simulink model "building_EXAMPLE_v1"  (R2016b)
settings: Solver=ode23tb  StartTime=-building.preruntime+8760*3600  StopTime=building.runtime+8760*3600  MaxStep=600  EnableMultiTasking=on
StartFcn:
  | tic
StopFcn:
  | toc
values from neighbouring files (symbols this model uses):
  building = create_building_automatic(building, modify, import_mode, name_XML, name_EXCEL, name_PHPP, NUMBEROFZONES)    [work_EXAMPLE_v1.m]
undefined symbols (not defined in the file or in its folder): A, B, C, cp, Dd, Dreifach, FluidMix, get_building, ID, MassFlow, p, Pressure, Qdot_C, Qdot_C_energy, Qdot_H, Qdot_H_energy, Qdot_I_electricity, Qdot_I_electricity_energy, Qdot_I_light, Qdot_I_light_energy, Qdot_I_person, Qdot_I_person_energy, Qdot_S, Qdot_S_energy, Qdot_T_ground, Qdot_T_ground_energy, Qdot_T_neighbour, Qdot_T_neighbour_energy, Qdot_T_opaque, Qdot_T_opaque_energy, Qdot_T_window, Qdot_T_window_energy, Qdot_V_infiltration, Qdot_V_infiltration_energy, Qdot_V_mech, Qdot_V_mech_energy, Qdot_V_window, Qdot_V_window_energy, rho, Tc, Temperature, Tr, Ts, Wärmeschutzglas, x_CO2, x_H2O, x_VOC
libraries: carnotUIBK x1931, carnot x83, simulink_extras x22, simulink x12
(part 12 of 35)

== system building_EXAMPLE_v1/HVAC pipes/ventilation_outlet1_z10 ==
  note: see energy balance
  note: no energy flux
  "[AIB]" : Inport
  Vdot : Inport  Port=2
  (kg/m³).(m³/h) : Product
  Bus Selector1 : BusSelector  OutputSignals=rho,Tc,p
  Bus Selector2 : BusSelector  OutputSignals=x_H2O
  Bus Selector3 : BusSelector  OutputSignals=x_CO2
  Fcn1 : Fcn  Expr=u / (1+u)
  Fcn2 : Fcn  Expr=u / (1+u)
  Gain : Gain  Gain=perc_Vdot_tot
  Gain1 : Gain  Gain=-1
  Gain3 : Gain  Gain=-1
  Gain4 : Gain  Gain=-1
  Ground{1..5} (5 alike) : Ground
  Mux1 : Mux  Inputs=[1 2 1 1 1 5 1 7]
  create_THB : Subsystem  mask(create THV){fluid=2, dia=0.125, hgt=0, mID=1}
      mask prompts: dia "diameter [m]"; hgt "Geodetic height in m"; mID "Calculation mode"
      mask help:
      | Create a THB with the variable input T and mdot. The other value can be set as constants in the mask.
      | Calculation mode:
      |     1 ..  9999 no pressure drop (dp)
      | 10001 .. 19999 dp caused by flowrate
      | 20001 .. inf   dp by flowrate and static height
      mask init:
      | dia = max(dia, 0.001);
      mask Help: web(fullfile(path_carnot('help'),'basic_create_THB.html'),'-helpbrowser')
  h/s : Gain  Gain=1/3600
  kg/s : Product
  kg/s1 : Product
  "[S]" : Outport
  THBout : Outport  Port=2  InitialOutput=0
  wires:
  create_THB/1(THB) -> THBout/1
  Bus Selector1/3 -> create_THB/3(p)  "<p>"
  Bus Selector1/2 -> create_THB/2(T)  "<Tc>"
  Vdot/1 -> Gain/1
  Ground3/1 -> Mux1/2
  Ground2/1 -> Mux1/8
  Ground1/1 -> Mux1/7
  Bus Selector3/1 -> Fcn1/1  "<x_CO2>"
  Bus Selector1/1 -> (kg/m³).(m³/h)/1  "<rho>"
  "[AIB]"/1 -> Bus Selector2/1, Bus Selector3/1, Bus Selector1/1
  Gain1/1 -> Mux1/5
  kg/s1/1 -> Gain1/1
  Fcn1/1 -> kg/s1/2
  Fcn2/1 -> kg/s/2
  Gain4/1 -> Mux1/3
  Ground5/1 -> Mux1/6
  Ground4/1 -> Mux1/1
  Gain3/1 -> Mux1/4
  kg/s/1 -> Gain3/1
  Bus Selector2/1 -> create_THB/4(mix), Fcn2/1  "<x_H2O>"
  h/s/1 -> Gain4/1, kg/s/1, create_THB/1(mdot), kg/s1/1
  (kg/m³).(m³/h)/1 -> h/s/1
  Gain/1 -> (kg/m³).(m³/h)/2
  Mux1/1 -> "[S]"/1

== system building_EXAMPLE_v1/HVAC pipes/ventilation_outlet1_z2 ==
  note: see energy balance
  note: no energy flux
  "[AIB]" : Inport
  Vdot : Inport  Port=2
  (kg/m³).(m³/h) : Product
  Bus Selector1 : BusSelector  OutputSignals=rho,Tc,p
  Bus Selector2 : BusSelector  OutputSignals=x_H2O
  Bus Selector3 : BusSelector  OutputSignals=x_CO2
  Fcn1 : Fcn  Expr=u / (1+u)
  Fcn2 : Fcn  Expr=u / (1+u)
  Gain : Gain  Gain=perc_Vdot_tot
  Gain1 : Gain  Gain=-1
  Gain3 : Gain  Gain=-1
  Gain4 : Gain  Gain=-1
  Ground{1..5} (5 alike) : Ground
  Mux1 : Mux  Inputs=[1 2 1 1 1 5 1 7]
  create_THB : Subsystem  mask(create THV){fluid=2, dia=0.125, hgt=0, mID=1}
      mask prompts: dia "diameter [m]"; hgt "Geodetic height in m"; mID "Calculation mode"
      mask help:
      | Create a THB with the variable input T and mdot. The other value can be set as constants in the mask.
      | Calculation mode:
      |     1 ..  9999 no pressure drop (dp)
      | 10001 .. 19999 dp caused by flowrate
      | 20001 .. inf   dp by flowrate and static height
      mask init:
      | dia = max(dia, 0.001);
      mask Help: web(fullfile(path_carnot('help'),'basic_create_THB.html'),'-helpbrowser')
  h/s : Gain  Gain=1/3600
  kg/s : Product
  kg/s1 : Product
  "[S]" : Outport
  THBout : Outport  Port=2  InitialOutput=0
  wires:
  create_THB/1(THB) -> THBout/1
  Bus Selector1/3 -> create_THB/3(p)  "<p>"
  Bus Selector1/2 -> create_THB/2(T)  "<Tc>"
  Vdot/1 -> Gain/1
  Ground3/1 -> Mux1/2
  Ground2/1 -> Mux1/8
  Ground1/1 -> Mux1/7
  Bus Selector3/1 -> Fcn1/1  "<x_CO2>"
  Bus Selector1/1 -> (kg/m³).(m³/h)/1  "<rho>"
  "[AIB]"/1 -> Bus Selector2/1, Bus Selector3/1, Bus Selector1/1
  Gain1/1 -> Mux1/5
  kg/s1/1 -> Gain1/1
  Fcn1/1 -> kg/s1/2
  Fcn2/1 -> kg/s/2
  Gain4/1 -> Mux1/3
  Ground5/1 -> Mux1/6
  Ground4/1 -> Mux1/1
  Gain3/1 -> Mux1/4
  kg/s/1 -> Gain3/1
  Bus Selector2/1 -> create_THB/4(mix), Fcn2/1  "<x_H2O>"
  h/s/1 -> Gain4/1, kg/s/1, create_THB/1(mdot), kg/s1/1
  (kg/m³).(m³/h)/1 -> h/s/1
  Gain/1 -> (kg/m³).(m³/h)/2
  Mux1/1 -> "[S]"/1

== system building_EXAMPLE_v1/HVAC pipes/ventilation_outlet1_z3 ==
  note: no energy flux
  note: see energy balance
  "[AIB]" : Inport
  Vdot : Inport  Port=2
  (kg/m³).(m³/h) : Product
  Bus Selector1 : BusSelector  OutputSignals=rho,Tc,p
  Bus Selector2 : BusSelector  OutputSignals=x_H2O
  Bus Selector3 : BusSelector  OutputSignals=x_CO2
  Fcn1 : Fcn  Expr=u / (1+u)
  Fcn2 : Fcn  Expr=u / (1+u)
  Gain : Gain  Gain=perc_Vdot_tot
  Gain1 : Gain  Gain=-1
  Gain3 : Gain  Gain=-1
  Gain4 : Gain  Gain=-1
  Ground{1..5} (5 alike) : Ground
  Mux1 : Mux  Inputs=[1 2 1 1 1 5 1 7]
  create_THB : Subsystem  mask(create THV){fluid=2, dia=0.125, hgt=0, mID=1}
      mask prompts: dia "diameter [m]"; hgt "Geodetic height in m"; mID "Calculation mode"
      mask help:
      | Create a THB with the variable input T and mdot. The other value can be set as constants in the mask.
      | Calculation mode:
      |     1 ..  9999 no pressure drop (dp)
      | 10001 .. 19999 dp caused by flowrate
      | 20001 .. inf   dp by flowrate and static height
      mask init:
      | dia = max(dia, 0.001);
      mask Help: web(fullfile(path_carnot('help'),'basic_create_THB.html'),'-helpbrowser')
  h/s : Gain  Gain=1/3600
  kg/s : Product
  kg/s1 : Product
  "[S]" : Outport
  THBout : Outport  Port=2  InitialOutput=0
  wires:
  Mux1/1 -> "[S]"/1
  Gain/1 -> (kg/m³).(m³/h)/2
  (kg/m³).(m³/h)/1 -> h/s/1
  h/s/1 -> create_THB/1(mdot), kg/s1/1, kg/s/1, Gain4/1
  Bus Selector2/1 -> create_THB/4(mix), Fcn2/1  "<x_H2O>"
  kg/s/1 -> Gain3/1
  Gain3/1 -> Mux1/4
  Ground4/1 -> Mux1/1
  Ground5/1 -> Mux1/6
  Gain4/1 -> Mux1/3
  Fcn2/1 -> kg/s/2
  Fcn1/1 -> kg/s1/2
  kg/s1/1 -> Gain1/1
  Gain1/1 -> Mux1/5
  "[AIB]"/1 -> Bus Selector1/1, Bus Selector3/1, Bus Selector2/1
  Bus Selector1/1 -> (kg/m³).(m³/h)/1  "<rho>"
  Bus Selector3/1 -> Fcn1/1  "<x_CO2>"
  Ground1/1 -> Mux1/7
  Ground2/1 -> Mux1/8
  Ground3/1 -> Mux1/2
  Vdot/1 -> Gain/1
  Bus Selector1/2 -> create_THB/2(T)  "<Tc>"
  Bus Selector1/3 -> create_THB/3(p)  "<p>"
  create_THB/1(THB) -> THBout/1

== system building_EXAMPLE_v1/HVAC pipes/ventilation_outlet1_z4 ==
  note: see energy balance
  note: no energy flux
  "[AIB]" : Inport
  Vdot : Inport  Port=2
  (kg/m³).(m³/h) : Product
  Bus Selector1 : BusSelector  OutputSignals=rho,Tc,p
  Bus Selector2 : BusSelector  OutputSignals=x_H2O
  Bus Selector3 : BusSelector  OutputSignals=x_CO2
  Fcn1 : Fcn  Expr=u / (1+u)
  Fcn2 : Fcn  Expr=u / (1+u)
  Gain : Gain  Gain=perc_Vdot_tot
  Gain1 : Gain  Gain=-1
  Gain3 : Gain  Gain=-1
  Gain4 : Gain  Gain=-1
  Ground{1..5} (5 alike) : Ground
  Mux1 : Mux  Inputs=[1 2 1 1 1 5 1 7]
  create_THB : Subsystem  mask(create THV){fluid=2, dia=0.125, hgt=0, mID=1}
      mask prompts: dia "diameter [m]"; hgt "Geodetic height in m"; mID "Calculation mode"
      mask help:
      | Create a THB with the variable input T and mdot. The other value can be set as constants in the mask.
      | Calculation mode:
      |     1 ..  9999 no pressure drop (dp)
      | 10001 .. 19999 dp caused by flowrate
      | 20001 .. inf   dp by flowrate and static height
      mask init:
      | dia = max(dia, 0.001);
      mask Help: web(fullfile(path_carnot('help'),'basic_create_THB.html'),'-helpbrowser')
  h/s : Gain  Gain=1/3600
  kg/s : Product
  kg/s1 : Product
  "[S]" : Outport
  THBout : Outport  Port=2  InitialOutput=0
  wires:
  create_THB/1(THB) -> THBout/1
  Bus Selector1/3 -> create_THB/3(p)  "<p>"
  Bus Selector1/2 -> create_THB/2(T)  "<Tc>"
  Vdot/1 -> Gain/1
  Ground3/1 -> Mux1/2
  Ground2/1 -> Mux1/8
  Ground1/1 -> Mux1/7
  Bus Selector3/1 -> Fcn1/1  "<x_CO2>"
  Bus Selector1/1 -> (kg/m³).(m³/h)/1  "<rho>"
  "[AIB]"/1 -> Bus Selector2/1, Bus Selector3/1, Bus Selector1/1
  Gain1/1 -> Mux1/5
  kg/s1/1 -> Gain1/1
  Fcn1/1 -> kg/s1/2
  Fcn2/1 -> kg/s/2
  Gain4/1 -> Mux1/3
  Ground5/1 -> Mux1/6
  Ground4/1 -> Mux1/1
  Gain3/1 -> Mux1/4
  kg/s/1 -> Gain3/1
  Bus Selector2/1 -> create_THB/4(mix), Fcn2/1  "<x_H2O>"
  h/s/1 -> Gain4/1, kg/s/1, create_THB/1(mdot), kg/s1/1
  (kg/m³).(m³/h)/1 -> h/s/1
  Gain/1 -> (kg/m³).(m³/h)/2
  Mux1/1 -> "[S]"/1

== system building_EXAMPLE_v1/HVAC pipes/ventilation_outlet1_z5 ==
  note: no energy flux
  note: see energy balance
  "[AIB]" : Inport
  Vdot : Inport  Port=2
  (kg/m³).(m³/h) : Product
  Bus Selector1 : BusSelector  OutputSignals=rho,Tc,p
  Bus Selector2 : BusSelector  OutputSignals=x_H2O
  Bus Selector3 : BusSelector  OutputSignals=x_CO2
  Fcn1 : Fcn  Expr=u / (1+u)
  Fcn2 : Fcn  Expr=u / (1+u)
  Gain : Gain  Gain=perc_Vdot_tot
  Gain1 : Gain  Gain=-1
  Gain3 : Gain  Gain=-1
  Gain4 : Gain  Gain=-1
  Ground{1..5} (5 alike) : Ground
  Mux1 : Mux  Inputs=[1 2 1 1 1 5 1 7]
  create_THB : Subsystem  mask(create THV){fluid=2, dia=0.125, hgt=0, mID=1}
      mask prompts: dia "diameter [m]"; hgt "Geodetic height in m"; mID "Calculation mode"
      mask help:
      | Create a THB with the variable input T and mdot. The other value can be set as constants in the mask.
      | Calculation mode:
      |     1 ..  9999 no pressure drop (dp)
      | 10001 .. 19999 dp caused by flowrate
      | 20001 .. inf   dp by flowrate and static height
      mask init:
      | dia = max(dia, 0.001);
      mask Help: web(fullfile(path_carnot('help'),'basic_create_THB.html'),'-helpbrowser')
  h/s : Gain  Gain=1/3600
  kg/s : Product
  kg/s1 : Product
  "[S]" : Outport
  THBout : Outport  Port=2  InitialOutput=0
  wires:
  Mux1/1 -> "[S]"/1
  Gain/1 -> (kg/m³).(m³/h)/2
  (kg/m³).(m³/h)/1 -> h/s/1
  h/s/1 -> create_THB/1(mdot), kg/s1/1, kg/s/1, Gain4/1
  Bus Selector2/1 -> create_THB/4(mix), Fcn2/1  "<x_H2O>"
  kg/s/1 -> Gain3/1
  Gain3/1 -> Mux1/4
  Ground4/1 -> Mux1/1
  Ground5/1 -> Mux1/6
  Gain4/1 -> Mux1/3
  Fcn2/1 -> kg/s/2
  Fcn1/1 -> kg/s1/2
  kg/s1/1 -> Gain1/1
  Gain1/1 -> Mux1/5
  "[AIB]"/1 -> Bus Selector1/1, Bus Selector3/1, Bus Selector2/1
  Bus Selector1/1 -> (kg/m³).(m³/h)/1  "<rho>"
  Bus Selector3/1 -> Fcn1/1  "<x_CO2>"
  Ground1/1 -> Mux1/7
  Ground2/1 -> Mux1/8
  Ground3/1 -> Mux1/2
  Vdot/1 -> Gain/1
  Bus Selector1/2 -> create_THB/2(T)  "<Tc>"
  Bus Selector1/3 -> create_THB/3(p)  "<p>"
  create_THB/1(THB) -> THBout/1

== system building_EXAMPLE_v1/HVAC pipes/ventilation_outlet1_z6 ==
  note: see energy balance
  note: no energy flux
  "[AIB]" : Inport
  Vdot : Inport  Port=2
  (kg/m³).(m³/h) : Product
  Bus Selector1 : BusSelector  OutputSignals=rho,Tc,p
  Bus Selector2 : BusSelector  OutputSignals=x_H2O
  Bus Selector3 : BusSelector  OutputSignals=x_CO2
  Fcn1 : Fcn  Expr=u / (1+u)
  Fcn2 : Fcn  Expr=u / (1+u)
  Gain : Gain  Gain=perc_Vdot_tot
  Gain1 : Gain  Gain=-1
  Gain3 : Gain  Gain=-1
  Gain4 : Gain  Gain=-1
  Ground{1..5} (5 alike) : Ground
  Mux1 : Mux  Inputs=[1 2 1 1 1 5 1 7]
  create_THB : Subsystem  mask(create THV){fluid=2, dia=0.125, hgt=0, mID=1}
      mask prompts: dia "diameter [m]"; hgt "Geodetic height in m"; mID "Calculation mode"
      mask help:
      | Create a THB with the variable input T and mdot. The other value can be set as constants in the mask.
      | Calculation mode:
      |     1 ..  9999 no pressure drop (dp)
      | 10001 .. 19999 dp caused by flowrate
      | 20001 .. inf   dp by flowrate and static height
      mask init:
      | dia = max(dia, 0.001);
      mask Help: web(fullfile(path_carnot('help'),'basic_create_THB.html'),'-helpbrowser')
  h/s : Gain  Gain=1/3600
  kg/s : Product
  kg/s1 : Product
  "[S]" : Outport
  THBout : Outport  Port=2  InitialOutput=0
  wires:
  create_THB/1(THB) -> THBout/1
  Bus Selector1/3 -> create_THB/3(p)  "<p>"
  Bus Selector1/2 -> create_THB/2(T)  "<Tc>"
  Vdot/1 -> Gain/1
  Ground3/1 -> Mux1/2
  Ground2/1 -> Mux1/8
  Ground1/1 -> Mux1/7
  Bus Selector3/1 -> Fcn1/1  "<x_CO2>"
  Bus Selector1/1 -> (kg/m³).(m³/h)/1  "<rho>"
  "[AIB]"/1 -> Bus Selector2/1, Bus Selector3/1, Bus Selector1/1
  Gain1/1 -> Mux1/5
  kg/s1/1 -> Gain1/1
  Fcn1/1 -> kg/s1/2
  Fcn2/1 -> kg/s/2
  Gain4/1 -> Mux1/3
  Ground5/1 -> Mux1/6
  Ground4/1 -> Mux1/1
  Gain3/1 -> Mux1/4
  kg/s/1 -> Gain3/1
  Bus Selector2/1 -> create_THB/4(mix), Fcn2/1  "<x_H2O>"
  h/s/1 -> Gain4/1, kg/s/1, create_THB/1(mdot), kg/s1/1
  (kg/m³).(m³/h)/1 -> h/s/1
  Gain/1 -> (kg/m³).(m³/h)/2
  Mux1/1 -> "[S]"/1

== system building_EXAMPLE_v1/HVAC pipes/ventilation_outlet1_z7 ==
  note: no energy flux
  note: see energy balance
  "[AIB]" : Inport
  Vdot : Inport  Port=2
  (kg/m³).(m³/h) : Product
  Bus Selector1 : BusSelector  OutputSignals=rho,Tc,p
  Bus Selector2 : BusSelector  OutputSignals=x_H2O
  Bus Selector3 : BusSelector  OutputSignals=x_CO2
  Fcn1 : Fcn  Expr=u / (1+u)
  Fcn2 : Fcn  Expr=u / (1+u)
  Gain : Gain  Gain=perc_Vdot_tot
  Gain1 : Gain  Gain=-1
  Gain3 : Gain  Gain=-1
  Gain4 : Gain  Gain=-1
  Ground{1..5} (5 alike) : Ground
  Mux1 : Mux  Inputs=[1 2 1 1 1 5 1 7]
  create_THB : Subsystem  mask(create THV){fluid=2, dia=0.125, hgt=0, mID=1}
      mask prompts: dia "diameter [m]"; hgt "Geodetic height in m"; mID "Calculation mode"
      mask help:
      | Create a THB with the variable input T and mdot. The other value can be set as constants in the mask.
      | Calculation mode:
      |     1 ..  9999 no pressure drop (dp)
      | 10001 .. 19999 dp caused by flowrate
      | 20001 .. inf   dp by flowrate and static height
      mask init:
      | dia = max(dia, 0.001);
      mask Help: web(fullfile(path_carnot('help'),'basic_create_THB.html'),'-helpbrowser')
  h/s : Gain  Gain=1/3600
  kg/s : Product
  kg/s1 : Product
  "[S]" : Outport
  THBout : Outport  Port=2  InitialOutput=0
  wires:
  Mux1/1 -> "[S]"/1
  Gain/1 -> (kg/m³).(m³/h)/2
  (kg/m³).(m³/h)/1 -> h/s/1
  h/s/1 -> create_THB/1(mdot), kg/s1/1, kg/s/1, Gain4/1
  Bus Selector2/1 -> create_THB/4(mix), Fcn2/1  "<x_H2O>"
  kg/s/1 -> Gain3/1
  Gain3/1 -> Mux1/4
  Ground4/1 -> Mux1/1
  Ground5/1 -> Mux1/6
  Gain4/1 -> Mux1/3
  Fcn2/1 -> kg/s/2
  Fcn1/1 -> kg/s1/2
  kg/s1/1 -> Gain1/1
  Gain1/1 -> Mux1/5
  "[AIB]"/1 -> Bus Selector1/1, Bus Selector3/1, Bus Selector2/1
  Bus Selector1/1 -> (kg/m³).(m³/h)/1  "<rho>"
  Bus Selector3/1 -> Fcn1/1  "<x_CO2>"
  Ground1/1 -> Mux1/7
  Ground2/1 -> Mux1/8
  Ground3/1 -> Mux1/2
  Vdot/1 -> Gain/1
  Bus Selector1/2 -> create_THB/2(T)  "<Tc>"
  Bus Selector1/3 -> create_THB/3(p)  "<p>"
  create_THB/1(THB) -> THBout/1

== system building_EXAMPLE_v1/HVAC pipes/ventilation_outlet1_z8 ==
  note: see energy balance
  note: no energy flux
  "[AIB]" : Inport
  Vdot : Inport  Port=2
  (kg/m³).(m³/h) : Product
  Bus Selector1 : BusSelector  OutputSignals=rho,Tc,p
  Bus Selector2 : BusSelector  OutputSignals=x_H2O
  Bus Selector3 : BusSelector  OutputSignals=x_CO2
  Fcn1 : Fcn  Expr=u / (1+u)
  Fcn2 : Fcn  Expr=u / (1+u)
  Gain : Gain  Gain=perc_Vdot_tot
  Gain1 : Gain  Gain=-1
  Gain3 : Gain  Gain=-1
  Gain4 : Gain  Gain=-1
  Ground{1..5} (5 alike) : Ground
  Mux1 : Mux  Inputs=[1 2 1 1 1 5 1 7]
  create_THB : Subsystem  mask(create THV){fluid=2, dia=0.125, hgt=0, mID=1}
      mask prompts: dia "diameter [m]"; hgt "Geodetic height in m"; mID "Calculation mode"
      mask help:
      | Create a THB with the variable input T and mdot. The other value can be set as constants in the mask.
      | Calculation mode:
      |     1 ..  9999 no pressure drop (dp)
      | 10001 .. 19999 dp caused by flowrate
      | 20001 .. inf   dp by flowrate and static height
      mask init:
      | dia = max(dia, 0.001);
      mask Help: web(fullfile(path_carnot('help'),'basic_create_THB.html'),'-helpbrowser')
  h/s : Gain  Gain=1/3600
  kg/s : Product
  kg/s1 : Product
  "[S]" : Outport
  THBout : Outport  Port=2  InitialOutput=0
  wires:
  create_THB/1(THB) -> THBout/1
  Bus Selector1/3 -> create_THB/3(p)  "<p>"
  Bus Selector1/2 -> create_THB/2(T)  "<Tc>"
  Vdot/1 -> Gain/1
  Ground3/1 -> Mux1/2
  Ground2/1 -> Mux1/8
  Ground1/1 -> Mux1/7
  Bus Selector3/1 -> Fcn1/1  "<x_CO2>"
  Bus Selector1/1 -> (kg/m³).(m³/h)/1  "<rho>"
  "[AIB]"/1 -> Bus Selector2/1, Bus Selector3/1, Bus Selector1/1
  Gain1/1 -> Mux1/5
  kg/s1/1 -> Gain1/1
  Fcn1/1 -> kg/s1/2
  Fcn2/1 -> kg/s/2
  Gain4/1 -> Mux1/3
  Ground5/1 -> Mux1/6
  Ground4/1 -> Mux1/1
  Gain3/1 -> Mux1/4
  kg/s/1 -> Gain3/1
  Bus Selector2/1 -> create_THB/4(mix), Fcn2/1  "<x_H2O>"
  h/s/1 -> Gain4/1, kg/s/1, create_THB/1(mdot), kg/s1/1
  (kg/m³).(m³/h)/1 -> h/s/1
  Gain/1 -> (kg/m³).(m³/h)/2
  Mux1/1 -> "[S]"/1

== system building_EXAMPLE_v1/HVAC pipes/ventilation_outlet1_z9 ==
  note: no energy flux
  note: see energy balance
  "[AIB]" : Inport
  Vdot : Inport  Port=2
  (kg/m³).(m³/h) : Product
  Bus Selector1 : BusSelector  OutputSignals=rho,Tc,p
  Bus Selector2 : BusSelector  OutputSignals=x_H2O
  Bus Selector3 : BusSelector  OutputSignals=x_CO2
  Fcn1 : Fcn  Expr=u / (1+u)
  Fcn2 : Fcn  Expr=u / (1+u)
  Gain : Gain  Gain=perc_Vdot_tot
  Gain1 : Gain  Gain=-1
  Gain3 : Gain  Gain=-1
  Gain4 : Gain  Gain=-1
  Ground{1..5} (5 alike) : Ground
  Mux1 : Mux  Inputs=[1 2 1 1 1 5 1 7]
  create_THB : Subsystem  mask(create THV){fluid=2, dia=0.125, hgt=0, mID=1}
      mask prompts: dia "diameter [m]"; hgt "Geodetic height in m"; mID "Calculation mode"
      mask help:
      | Create a THB with the variable input T and mdot. The other value can be set as constants in the mask.
      | Calculation mode:
      |     1 ..  9999 no pressure drop (dp)
      | 10001 .. 19999 dp caused by flowrate
      | 20001 .. inf   dp by flowrate and static height
      mask init:
      | dia = max(dia, 0.001);
      mask Help: web(fullfile(path_carnot('help'),'basic_create_THB.html'),'-helpbrowser')
  h/s : Gain  Gain=1/3600
  kg/s : Product
  kg/s1 : Product
  "[S]" : Outport
  THBout : Outport  Port=2  InitialOutput=0
  wires:
  Mux1/1 -> "[S]"/1
  Gain/1 -> (kg/m³).(m³/h)/2
  (kg/m³).(m³/h)/1 -> h/s/1
  h/s/1 -> create_THB/1(mdot), kg/s1/1, kg/s/1, Gain4/1
  Bus Selector2/1 -> create_THB/4(mix), Fcn2/1  "<x_H2O>"
  kg/s/1 -> Gain3/1
  Gain3/1 -> Mux1/4
  Ground4/1 -> Mux1/1
  Ground5/1 -> Mux1/6
  Gain4/1 -> Mux1/3
  Fcn2/1 -> kg/s/2
  Fcn1/1 -> kg/s1/2
  kg/s1/1 -> Gain1/1
  Gain1/1 -> Mux1/5
  "[AIB]"/1 -> Bus Selector1/1, Bus Selector3/1, Bus Selector2/1
  Bus Selector1/1 -> (kg/m³).(m³/h)/1  "<rho>"
  Bus Selector3/1 -> Fcn1/1  "<x_CO2>"
  Ground1/1 -> Mux1/7
  Ground2/1 -> Mux1/8
  Ground3/1 -> Mux1/2
  Vdot/1 -> Gain/1
  Bus Selector1/2 -> create_THB/2(T)  "<Tc>"
  Bus Selector1/3 -> create_THB/3(p)  "<p>"
  create_THB/1(THB) -> THBout/1

== system building_EXAMPLE_v1/HVAC pipes/ventilation_pipe_in_1 ==
  THBsupply : Inport
  Bus Selector : BusSelector  OutputSignals=MassFlow
  THB_set_mdot{1..10} (10 alike) : carnot/Source/Simple/THB_set_mdot
  zone_1 : Gain  Gain=hvac.zone(1).inlet(1)
  zone_10 : Gain  Gain=hvac.zone(10).inlet(1)
  zone_2 : Gain  Gain=hvac.zone(2).inlet(1)
  zone_3 : Gain  Gain=hvac.zone(3).inlet(1)
  zone_4 : Gain  Gain=hvac.zone(4).inlet(1)
  zone_5 : Gain  Gain=hvac.zone(5).inlet(1)
  zone_6 : Gain  Gain=hvac.zone(6).inlet(1)
  zone_7 : Gain  Gain=hvac.zone(7).inlet(1)
  zone_8 : Gain  Gain=hvac.zone(8).inlet(1)
  zone_9 : Gain  Gain=hvac.zone(9).inlet(1)
  "[TVBin_1]" : Outport
  "[TVBin_2]" : Outport  Port=2
  "[TVBin_3]" : Outport  Port=3
  "[TVBin_4]" : Outport  Port=4
  "[TVBin_5]" : Outport  Port=5
  "[TVBin_6]" : Outport  Port=6
  "[TVBin_7]" : Outport  Port=7
  "[TVBin_8]" : Outport  Port=8
  "[TVBin_9]" : Outport  Port=9
  "[TVBin_10]" : Outport  Port=10
  wires:
  THB_set_mdot1/1 -> "[TVBin_1]"/1
  THB_set_mdot2/1 -> "[TVBin_2]"/1
  Bus Selector/1 -> zone_3/1, zone_4/1, zone_5/1, zone_6/1, zone_7/1, zone_8/1, zone_9/1, zone_10/1, zone_2/1, zone_1/1  "<MassFlow>"
  zone_1/1 -> THB_set_mdot1/2
  zone_2/1 -> THB_set_mdot2/2
  THB_set_mdot5/1 -> "[TVBin_5]"/1
  THB_set_mdot4/1 -> "[TVBin_4]"/1
  THB_set_mdot3/1 -> "[TVBin_3]"/1
  THB_set_mdot6/1 -> "[TVBin_6]"/1
  THB_set_mdot7/1 -> "[TVBin_7]"/1
  THB_set_mdot8/1 -> "[TVBin_8]"/1
  THB_set_mdot9/1 -> "[TVBin_9]"/1
  THB_set_mdot10/1 -> "[TVBin_10]"/1
  THBsupply/1 -> Bus Selector/1, THB_set_mdot2/1, THB_set_mdot3/1, THB_set_mdot4/1, THB_set_mdot5/1, THB_set_mdot6/1, THB_set_mdot7/1, THB_set_mdot8/1, THB_set_mdot9/1, THB_set_mdot10/1, THB_set_mdot1/1
  zone_3/1 -> THB_set_mdot3/2
  zone_4/1 -> THB_set_mdot4/2
  zone_5/1 -> THB_set_mdot5/2
  zone_6/1 -> THB_set_mdot6/2
  zone_7/1 -> THB_set_mdot7/2
  zone_8/1 -> THB_set_mdot8/2
  zone_9/1 -> THB_set_mdot9/2
  zone_10/1 -> THB_set_mdot10/2

== system building_EXAMPLE_v1/HVAC pipes/ventilation_pipe_out_1 ==
  "[THBout_1]" : Inport
  "[THBout_2]" : Inport  Port=2
  "[THBout_3]" : Inport  Port=3
  "[THBout_4]" : Inport  Port=4
  "[THBout_5]" : Inport  Port=5
  "[THBout_6]" : Inport  Port=6
  "[THBout_7]" : Inport  Port=7
  "[THBout_8]" : Inport  Port=8
  "[THBout_9]" : Inport  Port=9
  "[THBout_10]" : Inport  Port=10
  mix : Subsystem
  mix1 : Subsystem
  mix2 : Subsystem
  mix3 : Subsystem
  mix4 : Subsystem
  mix5 : Subsystem
  mix6 : Subsystem
  mix7 : Subsystem
  mix8 : Subsystem
  THBextract : Outport
  wires:
  "[THBout_1]"/1 -> mix/1(THB_1)
  "[THBout_2]"/1 -> mix/2(THB_2)
  mix/1(THB) -> mix1/1(THB_1)
  "[THBout_3]"/1 -> mix1/2(THB_2)
  "[THBout_4]"/1 -> mix2/2(THB_2)
  mix1/1(THB) -> mix2/1(THB_1)
  mix2/1(THB) -> mix3/1(THB_1)
  mix3/1(THB) -> mix4/1(THB_1)
  mix4/1(THB) -> mix5/1(THB_1)
  mix5/1(THB) -> mix6/1(THB_1)
  "[THBout_5]"/1 -> mix3/2(THB_2)
  "[THBout_6]"/1 -> mix4/2(THB_2)
  "[THBout_7]"/1 -> mix5/2(THB_2)
  "[THBout_8]"/1 -> mix6/2(THB_2)
  mix6/1(THB) -> mix7/1(THB_1)
  mix7/1(THB) -> mix8/1(THB_1)
  mix8/1(THB) -> THBextract/1
  "[THBout_10]"/1 -> mix8/2(THB_2)
  "[THBout_9]"/1 -> mix7/2(THB_2)

== system building_EXAMPLE_v1/HVAC pipes/ventilation_zone-to-zone 1-10 ==
  "[AIB]_in" : Inport
  "[AIB]_out" : Inport  Port=2
  Vdot : Inport  Port=3
  Bus Selector1 : BusSelector  OutputSignals=Tc,x_H2O,x_CO2,rho
  Bus Selector2 : BusSelector  OutputSignals=Tc,x_H2O,x_CO2,rho
  Demux5 : Demux  Outputs=2
  Fcn{1..4} (4 alike) : Fcn  Expr=u / (1+u)
  Gain : Gain  Gain=perc_Vdot_tot
  Gain{1,4..5,7} (4 alike) : Gain  Gain=-1
  Gain2 : Gain  Gain=0
  Ground{1..6,12..13} (8 alike) : Ground
  Mux1 : Mux  Inputs=[1 2 1 1 1 5 1 7]
  Mux2 : Mux  Inputs=[1 2 1 1 1 5 1 7]
  Mux3 : Mux  Inputs=2
  Mux6 : Mux  Inputs=2
  Product5 : Product  SaturateOnIntegerOverflow=on  InputSameDT=on  OutDataTypeStr=Inherit: Same as first input
  Product6 : Product  SaturateOnIntegerOverflow=on  InputSameDT=on  OutDataTypeStr=Inherit: Same as first input
  Product7 : Product  Inputs=3  SaturateOnIntegerOverflow=on  InputSameDT=on  OutDataTypeStr=Inherit: Same as first input
  Sum1 : Sum  Inputs=-+  SaturateOnIntegerOverflow=on  InputSameDT=on  OutDataTypeStr=Inherit: Same as first input
  Switch : Switch  Criteria=u2 > Threshold
  Switch1 : Switch  Criteria=u2 > Threshold
  cp : Constant  Value=1006.8
  h/s : Gain  Gain=1/3600
  "[S]_in" : Outport
  "[S]_out" : Outport  Port=2
  wires:
  Mux3/1 -> Switch1/1
  Mux6/1 -> Switch1/3
  Bus Selector1/3 -> Fcn3/1  "<x_CO2>"
  Bus Selector1/2 -> Fcn4/1  "<x_H2O>"
  Fcn3/1 -> Mux3/2
  Fcn4/1 -> Mux3/1
  Bus Selector2/4 -> Switch/3  "<rho>"
  Bus Selector1/4 -> Switch/1  "<rho>"
  "[AIB]_in"/1 -> Bus Selector1/1
  cp/1 -> Product7/3
  Ground4/1 -> Mux1/7
  Ground1/1 -> Mux1/8
  "[AIB]_out"/1 -> Bus Selector2/1
  Bus Selector1/1 -> Sum1/1  "<Tc>"
  Fcn1/1 -> Mux6/2
  Fcn2/1 -> Mux6/1
  Ground12/1 -> Mux1/6
  Product5/1 -> Demux5/1
  Bus Selector2/3 -> Fcn1/1  "<x_CO2>"
  Mux2/1 -> "[S]_out"/1
  Switch/1 -> Product6/2  "rho"
  Product6/1 -> Gain1/1
  Gain/1 -> Switch/2, Switch1/2, h/s/1
  Mux1/1 -> "[S]_in"/1
  Product7/1 -> Gain2/1, Mux1/1  "Qdot_air"
  Ground13/1 -> Mux1/2
  Demux5/2 -> Mux1/5, Gain5/1  "mdot_CO2"
  Demux5/1 -> Mux1/4, Gain4/1  "mdot_H2O"
  Bus Selector2/1 -> Sum1/2  "<Tc>"
  Bus Selector2/2 -> Fcn2/1  "<x_H2O>"
  Switch1/1 -> Product5/2
  Sum1/1 -> Product7/1  "dT"
  Vdot/1 -> Gain/1
  h/s/1 -> Product6/1
  Gain1/1 -> Gain7/1, Product5/1, Product7/2, Mux1/3  "massflow"
  Ground3/1 -> Mux2/7
  Gain4/1 -> Mux2/4
  Gain7/1 -> Mux2/3
  Ground2/1 -> Mux2/2
  Gain5/1 -> Mux2/5
  Ground5/1 -> Mux2/6
  Ground6/1 -> Mux2/8
  Gain2/1 -> Mux2/1

== system building_EXAMPLE_v1/HVAC pipes/ventilation_zone-to-zone 1-2 ==
  "[AIB]_in" : Inport
  "[AIB]_out" : Inport  Port=2
  Vdot : Inport  Port=3
  Bus Selector1 : BusSelector  OutputSignals=Tc,x_H2O,x_CO2,rho
  Bus Selector2 : BusSelector  OutputSignals=Tc,x_H2O,x_CO2,rho
  Demux5 : Demux  Outputs=2
  Fcn{1..4} (4 alike) : Fcn  Expr=u / (1+u)
  Gain : Gain  Gain=perc_Vdot_tot
  Gain{1,4..5,7} (4 alike) : Gain  Gain=-1
  Gain2 : Gain  Gain=0
  Ground{1..6,12..13} (8 alike) : Ground
  Mux1 : Mux  Inputs=[1 2 1 1 1 5 1 7]
  Mux2 : Mux  Inputs=[1 2 1 1 1 5 1 7]
  Mux3 : Mux  Inputs=2
  Mux6 : Mux  Inputs=2
  Product5 : Product  SaturateOnIntegerOverflow=on  InputSameDT=on  OutDataTypeStr=Inherit: Same as first input
  Product6 : Product  SaturateOnIntegerOverflow=on  InputSameDT=on  OutDataTypeStr=Inherit: Same as first input
  Product7 : Product  Inputs=3  SaturateOnIntegerOverflow=on  InputSameDT=on  OutDataTypeStr=Inherit: Same as first input
  Sum1 : Sum  Inputs=-+  SaturateOnIntegerOverflow=on  InputSameDT=on  OutDataTypeStr=Inherit: Same as first input
  Switch : Switch  Criteria=u2 > Threshold
  Switch1 : Switch  Criteria=u2 > Threshold
  cp : Constant  Value=1006.8
  h/s : Gain  Gain=1/3600
  "[S]_in" : Outport
  "[S]_out" : Outport  Port=2
  wires:
  Mux3/1 -> Switch1/1
  Mux6/1 -> Switch1/3
  Bus Selector1/3 -> Fcn3/1  "<x_CO2>"
  Bus Selector1/2 -> Fcn4/1  "<x_H2O>"
  Fcn3/1 -> Mux3/2
  Fcn4/1 -> Mux3/1
  Bus Selector2/4 -> Switch/3  "<rho>"
  Bus Selector1/4 -> Switch/1  "<rho>"
  "[AIB]_in"/1 -> Bus Selector1/1
  cp/1 -> Product7/3
  Ground4/1 -> Mux1/7
  Ground1/1 -> Mux1/8
  "[AIB]_out"/1 -> Bus Selector2/1
  Bus Selector1/1 -> Sum1/1  "<Tc>"
  Fcn1/1 -> Mux6/2
  Fcn2/1 -> Mux6/1
  Ground12/1 -> Mux1/6
  Product5/1 -> Demux5/1
  Bus Selector2/3 -> Fcn1/1  "<x_CO2>"
  Mux2/1 -> "[S]_out"/1
  Switch/1 -> Product6/2  "rho"
  Product6/1 -> Gain1/1
  Gain/1 -> Switch/2, Switch1/2, h/s/1
  Mux1/1 -> "[S]_in"/1
  Product7/1 -> Gain2/1, Mux1/1  "Qdot_air"
  Ground13/1 -> Mux1/2
  Demux5/2 -> Mux1/5, Gain5/1  "mdot_CO2"
  Demux5/1 -> Mux1/4, Gain4/1  "mdot_H2O"
  Bus Selector2/1 -> Sum1/2  "<Tc>"
  Bus Selector2/2 -> Fcn2/1  "<x_H2O>"
  Switch1/1 -> Product5/2
  Sum1/1 -> Product7/1  "dT"
  Vdot/1 -> Gain/1
  h/s/1 -> Product6/1
  Gain1/1 -> Gain7/1, Product5/1, Product7/2, Mux1/3  "massflow"
  Ground3/1 -> Mux2/7
  Gain4/1 -> Mux2/4
  Gain7/1 -> Mux2/3
  Ground2/1 -> Mux2/2
  Gain5/1 -> Mux2/5
  Ground5/1 -> Mux2/6
  Ground6/1 -> Mux2/8
  Gain2/1 -> Mux2/1

== system building_EXAMPLE_v1/HVAC pipes/ventilation_zone-to-zone 1-3 ==
  "[AIB]_in" : Inport
  "[AIB]_out" : Inport  Port=2
  Vdot : Inport  Port=3
  Bus Selector1 : BusSelector  OutputSignals=Tc,x_H2O,x_CO2,rho
  Bus Selector2 : BusSelector  OutputSignals=Tc,x_H2O,x_CO2,rho
  Demux5 : Demux  Outputs=2
  Fcn{1..4} (4 alike) : Fcn  Expr=u / (1+u)
  Gain : Gain  Gain=perc_Vdot_tot
  Gain{1,4..5,7} (4 alike) : Gain  Gain=-1
  Gain2 : Gain  Gain=0
  Ground{1..6,12..13} (8 alike) : Ground
  Mux1 : Mux  Inputs=[1 2 1 1 1 5 1 7]
  Mux2 : Mux  Inputs=[1 2 1 1 1 5 1 7]
  Mux3 : Mux  Inputs=2
  Mux6 : Mux  Inputs=2
  Product5 : Product  SaturateOnIntegerOverflow=on  InputSameDT=on  OutDataTypeStr=Inherit: Same as first input
  Product6 : Product  SaturateOnIntegerOverflow=on  InputSameDT=on  OutDataTypeStr=Inherit: Same as first input
  Product7 : Product  Inputs=3  SaturateOnIntegerOverflow=on  InputSameDT=on  OutDataTypeStr=Inherit: Same as first input
  Sum1 : Sum  Inputs=-+  SaturateOnIntegerOverflow=on  InputSameDT=on  OutDataTypeStr=Inherit: Same as first input
  Switch : Switch  Criteria=u2 > Threshold
  Switch1 : Switch  Criteria=u2 > Threshold
  cp : Constant  Value=1006.8
  h/s : Gain  Gain=1/3600
  "[S]_in" : Outport
  "[S]_out" : Outport  Port=2
  wires:
  Mux3/1 -> Switch1/1
  Mux6/1 -> Switch1/3
  Bus Selector1/3 -> Fcn3/1  "<x_CO2>"
  Bus Selector1/2 -> Fcn4/1  "<x_H2O>"
  Fcn3/1 -> Mux3/2
  Fcn4/1 -> Mux3/1
  Bus Selector2/4 -> Switch/3  "<rho>"
  Bus Selector1/4 -> Switch/1  "<rho>"
  "[AIB]_in"/1 -> Bus Selector1/1
  cp/1 -> Product7/3
  Ground4/1 -> Mux1/7
  Ground1/1 -> Mux1/8
  "[AIB]_out"/1 -> Bus Selector2/1
  Bus Selector1/1 -> Sum1/1  "<Tc>"
  Fcn1/1 -> Mux6/2
  Fcn2/1 -> Mux6/1
  Ground12/1 -> Mux1/6
  Product5/1 -> Demux5/1
  Bus Selector2/3 -> Fcn1/1  "<x_CO2>"
  Mux2/1 -> "[S]_out"/1
  Switch/1 -> Product6/2  "rho"
  Product6/1 -> Gain1/1
  Gain/1 -> Switch/2, Switch1/2, h/s/1
  Mux1/1 -> "[S]_in"/1
  Product7/1 -> Gain2/1, Mux1/1  "Qdot_air"
  Ground13/1 -> Mux1/2
  Demux5/2 -> Mux1/5, Gain5/1  "mdot_CO2"
  Demux5/1 -> Mux1/4, Gain4/1  "mdot_H2O"
  Bus Selector2/1 -> Sum1/2  "<Tc>"
  Bus Selector2/2 -> Fcn2/1  "<x_H2O>"
  Switch1/1 -> Product5/2
  Sum1/1 -> Product7/1  "dT"
  Vdot/1 -> Gain/1
  h/s/1 -> Product6/1
  Gain1/1 -> Gain7/1, Product5/1, Product7/2, Mux1/3  "massflow"
  Ground3/1 -> Mux2/7
  Gain4/1 -> Mux2/4
  Gain7/1 -> Mux2/3
  Ground2/1 -> Mux2/2
  Gain5/1 -> Mux2/5
  Ground5/1 -> Mux2/6
  Ground6/1 -> Mux2/8
  Gain2/1 -> Mux2/1

== system building_EXAMPLE_v1/HVAC pipes/ventilation_zone-to-zone 1-4 ==
  "[AIB]_in" : Inport
  "[AIB]_out" : Inport  Port=2
  Vdot : Inport  Port=3
  Bus Selector1 : BusSelector  OutputSignals=Tc,x_H2O,x_CO2,rho
  Bus Selector2 : BusSelector  OutputSignals=Tc,x_H2O,x_CO2,rho
  Demux5 : Demux  Outputs=2
  Fcn{1..4} (4 alike) : Fcn  Expr=u / (1+u)
  Gain : Gain  Gain=perc_Vdot_tot
  Gain{1,4..5,7} (4 alike) : Gain  Gain=-1
  Gain2 : Gain  Gain=0
  Ground{1..6,12..13} (8 alike) : Ground
  Mux1 : Mux  Inputs=[1 2 1 1 1 5 1 7]
  Mux2 : Mux  Inputs=[1 2 1 1 1 5 1 7]
  Mux3 : Mux  Inputs=2
  Mux6 : Mux  Inputs=2
  Product5 : Product  SaturateOnIntegerOverflow=on  InputSameDT=on  OutDataTypeStr=Inherit: Same as first input
  Product6 : Product  SaturateOnIntegerOverflow=on  InputSameDT=on  OutDataTypeStr=Inherit: Same as first input
  Product7 : Product  Inputs=3  SaturateOnIntegerOverflow=on  InputSameDT=on  OutDataTypeStr=Inherit: Same as first input
  Sum1 : Sum  Inputs=-+  SaturateOnIntegerOverflow=on  InputSameDT=on  OutDataTypeStr=Inherit: Same as first input
  Switch : Switch  Criteria=u2 > Threshold
  Switch1 : Switch  Criteria=u2 > Threshold
  cp : Constant  Value=1006.8
  h/s : Gain  Gain=1/3600
  "[S]_in" : Outport
  "[S]_out" : Outport  Port=2
  wires:
  Mux3/1 -> Switch1/1
  Mux6/1 -> Switch1/3
  Bus Selector1/3 -> Fcn3/1  "<x_CO2>"
  Bus Selector1/2 -> Fcn4/1  "<x_H2O>"
  Fcn3/1 -> Mux3/2
  Fcn4/1 -> Mux3/1
  Bus Selector2/4 -> Switch/3  "<rho>"
  Bus Selector1/4 -> Switch/1  "<rho>"
  "[AIB]_in"/1 -> Bus Selector1/1
  cp/1 -> Product7/3
  Ground4/1 -> Mux1/7
  Ground1/1 -> Mux1/8
  "[AIB]_out"/1 -> Bus Selector2/1
  Bus Selector1/1 -> Sum1/1  "<Tc>"
  Fcn1/1 -> Mux6/2
  Fcn2/1 -> Mux6/1
  Ground12/1 -> Mux1/6
  Product5/1 -> Demux5/1
  Bus Selector2/3 -> Fcn1/1  "<x_CO2>"
  Mux2/1 -> "[S]_out"/1
  Switch/1 -> Product6/2  "rho"
  Product6/1 -> Gain1/1
  Gain/1 -> Switch/2, Switch1/2, h/s/1
  Mux1/1 -> "[S]_in"/1
  Product7/1 -> Gain2/1, Mux1/1  "Qdot_air"
  Ground13/1 -> Mux1/2
  Demux5/2 -> Mux1/5, Gain5/1  "mdot_CO2"
  Demux5/1 -> Mux1/4, Gain4/1  "mdot_H2O"
  Bus Selector2/1 -> Sum1/2  "<Tc>"
  Bus Selector2/2 -> Fcn2/1  "<x_H2O>"
  Switch1/1 -> Product5/2
  Sum1/1 -> Product7/1  "dT"
  Vdot/1 -> Gain/1
  h/s/1 -> Product6/1
  Gain1/1 -> Gain7/1, Product5/1, Product7/2, Mux1/3  "massflow"
  Ground3/1 -> Mux2/7
  Gain4/1 -> Mux2/4
  Gain7/1 -> Mux2/3
  Ground2/1 -> Mux2/2
  Gain5/1 -> Mux2/5
  Ground5/1 -> Mux2/6
  Ground6/1 -> Mux2/8
  Gain2/1 -> Mux2/1

== system building_EXAMPLE_v1/HVAC pipes/ventilation_zone-to-zone 1-5 ==
  "[AIB]_in" : Inport
  "[AIB]_out" : Inport  Port=2
  Vdot : Inport  Port=3
  Bus Selector1 : BusSelector  OutputSignals=Tc,x_H2O,x_CO2,rho
  Bus Selector2 : BusSelector  OutputSignals=Tc,x_H2O,x_CO2,rho
  Demux5 : Demux  Outputs=2
  Fcn{1..4} (4 alike) : Fcn  Expr=u / (1+u)
  Gain : Gain  Gain=perc_Vdot_tot
  Gain{1,4..5,7} (4 alike) : Gain  Gain=-1
  Gain2 : Gain  Gain=0
  Ground{1..6,12..13} (8 alike) : Ground
  Mux1 : Mux  Inputs=[1 2 1 1 1 5 1 7]
  Mux2 : Mux  Inputs=[1 2 1 1 1 5 1 7]
  Mux3 : Mux  Inputs=2
  Mux6 : Mux  Inputs=2
  Product5 : Product  SaturateOnIntegerOverflow=on  InputSameDT=on  OutDataTypeStr=Inherit: Same as first input
  Product6 : Product  SaturateOnIntegerOverflow=on  InputSameDT=on  OutDataTypeStr=Inherit: Same as first input
  Product7 : Product  Inputs=3  SaturateOnIntegerOverflow=on  InputSameDT=on  OutDataTypeStr=Inherit: Same as first input
  Sum1 : Sum  Inputs=-+  SaturateOnIntegerOverflow=on  InputSameDT=on  OutDataTypeStr=Inherit: Same as first input
  Switch : Switch  Criteria=u2 > Threshold
  Switch1 : Switch  Criteria=u2 > Threshold
  cp : Constant  Value=1006.8
  h/s : Gain  Gain=1/3600
  "[S]_in" : Outport
  "[S]_out" : Outport  Port=2
  wires:
  Mux3/1 -> Switch1/1
  Mux6/1 -> Switch1/3
  Bus Selector1/3 -> Fcn3/1  "<x_CO2>"
  Bus Selector1/2 -> Fcn4/1  "<x_H2O>"
  Fcn3/1 -> Mux3/2
  Fcn4/1 -> Mux3/1
  Bus Selector2/4 -> Switch/3  "<rho>"
  Bus Selector1/4 -> Switch/1  "<rho>"
  "[AIB]_in"/1 -> Bus Selector1/1
  cp/1 -> Product7/3
  Ground4/1 -> Mux1/7
  Ground1/1 -> Mux1/8
  "[AIB]_out"/1 -> Bus Selector2/1
  Bus Selector1/1 -> Sum1/1  "<Tc>"
  Fcn1/1 -> Mux6/2
  Fcn2/1 -> Mux6/1
  Ground12/1 -> Mux1/6
  Product5/1 -> Demux5/1
  Bus Selector2/3 -> Fcn1/1  "<x_CO2>"
  Mux2/1 -> "[S]_out"/1
  Switch/1 -> Product6/2  "rho"
  Product6/1 -> Gain1/1
  Gain/1 -> Switch/2, Switch1/2, h/s/1
  Mux1/1 -> "[S]_in"/1
  Product7/1 -> Gain2/1, Mux1/1  "Qdot_air"
  Ground13/1 -> Mux1/2
  Demux5/2 -> Mux1/5, Gain5/1  "mdot_CO2"
  Demux5/1 -> Mux1/4, Gain4/1  "mdot_H2O"
  Bus Selector2/1 -> Sum1/2  "<Tc>"
  Bus Selector2/2 -> Fcn2/1  "<x_H2O>"
  Switch1/1 -> Product5/2
  Sum1/1 -> Product7/1  "dT"
  Vdot/1 -> Gain/1
  h/s/1 -> Product6/1
  Gain1/1 -> Gain7/1, Product5/1, Product7/2, Mux1/3  "massflow"
  Ground3/1 -> Mux2/7
  Gain4/1 -> Mux2/4
  Gain7/1 -> Mux2/3
  Ground2/1 -> Mux2/2
  Gain5/1 -> Mux2/5
  Ground5/1 -> Mux2/6
  Ground6/1 -> Mux2/8
  Gain2/1 -> Mux2/1

== system building_EXAMPLE_v1/HVAC pipes/ventilation_zone-to-zone 1-6 ==
  "[AIB]_in" : Inport
  "[AIB]_out" : Inport  Port=2
  Vdot : Inport  Port=3
  Bus Selector1 : BusSelector  OutputSignals=Tc,x_H2O,x_CO2,rho
  Bus Selector2 : BusSelector  OutputSignals=Tc,x_H2O,x_CO2,rho
  Demux5 : Demux  Outputs=2
  Fcn{1..4} (4 alike) : Fcn  Expr=u / (1+u)
  Gain : Gain  Gain=perc_Vdot_tot
  Gain{1,4..5,7} (4 alike) : Gain  Gain=-1
  Gain2 : Gain  Gain=0
  Ground{1..6,12..13} (8 alike) : Ground
  Mux1 : Mux  Inputs=[1 2 1 1 1 5 1 7]
  Mux2 : Mux  Inputs=[1 2 1 1 1 5 1 7]
  Mux3 : Mux  Inputs=2
  Mux6 : Mux  Inputs=2
  Product5 : Product  SaturateOnIntegerOverflow=on  InputSameDT=on  OutDataTypeStr=Inherit: Same as first input
  Product6 : Product  SaturateOnIntegerOverflow=on  InputSameDT=on  OutDataTypeStr=Inherit: Same as first input
  Product7 : Product  Inputs=3  SaturateOnIntegerOverflow=on  InputSameDT=on  OutDataTypeStr=Inherit: Same as first input
  Sum1 : Sum  Inputs=-+  SaturateOnIntegerOverflow=on  InputSameDT=on  OutDataTypeStr=Inherit: Same as first input
  Switch : Switch  Criteria=u2 > Threshold
  Switch1 : Switch  Criteria=u2 > Threshold
  cp : Constant  Value=1006.8
  h/s : Gain  Gain=1/3600
  "[S]_in" : Outport
  "[S]_out" : Outport  Port=2
  wires:
  Mux3/1 -> Switch1/1
  Mux6/1 -> Switch1/3
  Bus Selector1/3 -> Fcn3/1  "<x_CO2>"
  Bus Selector1/2 -> Fcn4/1  "<x_H2O>"
  Fcn3/1 -> Mux3/2
  Fcn4/1 -> Mux3/1
  Bus Selector2/4 -> Switch/3  "<rho>"
  Bus Selector1/4 -> Switch/1  "<rho>"
  "[AIB]_in"/1 -> Bus Selector1/1
  cp/1 -> Product7/3
  Ground4/1 -> Mux1/7
  Ground1/1 -> Mux1/8
  "[AIB]_out"/1 -> Bus Selector2/1
  Bus Selector1/1 -> Sum1/1  "<Tc>"
  Fcn1/1 -> Mux6/2
  Fcn2/1 -> Mux6/1
  Ground12/1 -> Mux1/6
  Product5/1 -> Demux5/1
  Bus Selector2/3 -> Fcn1/1  "<x_CO2>"
  Mux2/1 -> "[S]_out"/1
  Switch/1 -> Product6/2  "rho"
  Product6/1 -> Gain1/1
  Gain/1 -> Switch/2, Switch1/2, h/s/1
  Mux1/1 -> "[S]_in"/1
  Product7/1 -> Gain2/1, Mux1/1  "Qdot_air"
  Ground13/1 -> Mux1/2
  Demux5/2 -> Mux1/5, Gain5/1  "mdot_CO2"
  Demux5/1 -> Mux1/4, Gain4/1  "mdot_H2O"
  Bus Selector2/1 -> Sum1/2  "<Tc>"
  Bus Selector2/2 -> Fcn2/1  "<x_H2O>"
  Switch1/1 -> Product5/2
  Sum1/1 -> Product7/1  "dT"
  Vdot/1 -> Gain/1
  h/s/1 -> Product6/1
  Gain1/1 -> Gain7/1, Product5/1, Product7/2, Mux1/3  "massflow"
  Ground3/1 -> Mux2/7
  Gain4/1 -> Mux2/4
  Gain7/1 -> Mux2/3
  Ground2/1 -> Mux2/2
  Gain5/1 -> Mux2/5
  Ground5/1 -> Mux2/6
  Ground6/1 -> Mux2/8
  Gain2/1 -> Mux2/1

== system building_EXAMPLE_v1/HVAC pipes/ventilation_zone-to-zone 1-7 ==
  "[AIB]_in" : Inport
  "[AIB]_out" : Inport  Port=2
  Vdot : Inport  Port=3
  Bus Selector1 : BusSelector  OutputSignals=Tc,x_H2O,x_CO2,rho
  Bus Selector2 : BusSelector  OutputSignals=Tc,x_H2O,x_CO2,rho
  Demux5 : Demux  Outputs=2
  Fcn{1..4} (4 alike) : Fcn  Expr=u / (1+u)
  Gain : Gain  Gain=perc_Vdot_tot
  Gain{1,4..5,7} (4 alike) : Gain  Gain=-1
  Gain2 : Gain  Gain=0
  Ground{1..6,12..13} (8 alike) : Ground
  Mux1 : Mux  Inputs=[1 2 1 1 1 5 1 7]
  Mux2 : Mux  Inputs=[1 2 1 1 1 5 1 7]
  Mux3 : Mux  Inputs=2
  Mux6 : Mux  Inputs=2
  Product5 : Product  SaturateOnIntegerOverflow=on  InputSameDT=on  OutDataTypeStr=Inherit: Same as first input
  Product6 : Product  SaturateOnIntegerOverflow=on  InputSameDT=on  OutDataTypeStr=Inherit: Same as first input
  Product7 : Product  Inputs=3  SaturateOnIntegerOverflow=on  InputSameDT=on  OutDataTypeStr=Inherit: Same as first input
  Sum1 : Sum  Inputs=-+  SaturateOnIntegerOverflow=on  InputSameDT=on  OutDataTypeStr=Inherit: Same as first input
  Switch : Switch  Criteria=u2 > Threshold
  Switch1 : Switch  Criteria=u2 > Threshold
  cp : Constant  Value=1006.8
  h/s : Gain  Gain=1/3600
  "[S]_in" : Outport
  "[S]_out" : Outport  Port=2
  wires:
  Mux3/1 -> Switch1/1
  Mux6/1 -> Switch1/3
  Bus Selector1/3 -> Fcn3/1  "<x_CO2>"
  Bus Selector1/2 -> Fcn4/1  "<x_H2O>"
  Fcn3/1 -> Mux3/2
  Fcn4/1 -> Mux3/1
  Bus Selector2/4 -> Switch/3  "<rho>"
  Bus Selector1/4 -> Switch/1  "<rho>"
  "[AIB]_in"/1 -> Bus Selector1/1
  cp/1 -> Product7/3
  Ground4/1 -> Mux1/7
  Ground1/1 -> Mux1/8
  "[AIB]_out"/1 -> Bus Selector2/1
  Bus Selector1/1 -> Sum1/1  "<Tc>"
  Fcn1/1 -> Mux6/2
  Fcn2/1 -> Mux6/1
  Ground12/1 -> Mux1/6
  Product5/1 -> Demux5/1
  Bus Selector2/3 -> Fcn1/1  "<x_CO2>"
  Mux2/1 -> "[S]_out"/1
  Switch/1 -> Product6/2  "rho"
  Product6/1 -> Gain1/1
  Gain/1 -> Switch/2, Switch1/2, h/s/1
  Mux1/1 -> "[S]_in"/1
  Product7/1 -> Gain2/1, Mux1/1  "Qdot_air"
  Ground13/1 -> Mux1/2
  Demux5/2 -> Mux1/5, Gain5/1  "mdot_CO2"
  Demux5/1 -> Mux1/4, Gain4/1  "mdot_H2O"
  Bus Selector2/1 -> Sum1/2  "<Tc>"
  Bus Selector2/2 -> Fcn2/1  "<x_H2O>"
  Switch1/1 -> Product5/2
  Sum1/1 -> Product7/1  "dT"
  Vdot/1 -> Gain/1
  h/s/1 -> Product6/1
  Gain1/1 -> Gain7/1, Product5/1, Product7/2, Mux1/3  "massflow"
  Ground3/1 -> Mux2/7
  Gain4/1 -> Mux2/4
  Gain7/1 -> Mux2/3
  Ground2/1 -> Mux2/2
  Gain5/1 -> Mux2/5
  Ground5/1 -> Mux2/6
  Ground6/1 -> Mux2/8
  Gain2/1 -> Mux2/1

== system building_EXAMPLE_v1/HVAC pipes/ventilation_zone-to-zone 1-8 ==
  "[AIB]_in" : Inport
  "[AIB]_out" : Inport  Port=2
  Vdot : Inport  Port=3
  Bus Selector1 : BusSelector  OutputSignals=Tc,x_H2O,x_CO2,rho
  Bus Selector2 : BusSelector  OutputSignals=Tc,x_H2O,x_CO2,rho
  Demux5 : Demux  Outputs=2
  Fcn{1..4} (4 alike) : Fcn  Expr=u / (1+u)
  Gain : Gain  Gain=perc_Vdot_tot
  Gain{1,4..5,7} (4 alike) : Gain  Gain=-1
  Gain2 : Gain  Gain=0
  Ground{1..6,12..13} (8 alike) : Ground
  Mux1 : Mux  Inputs=[1 2 1 1 1 5 1 7]
  Mux2 : Mux  Inputs=[1 2 1 1 1 5 1 7]
  Mux3 : Mux  Inputs=2
  Mux6 : Mux  Inputs=2
  Product5 : Product  SaturateOnIntegerOverflow=on  InputSameDT=on  OutDataTypeStr=Inherit: Same as first input
  Product6 : Product  SaturateOnIntegerOverflow=on  InputSameDT=on  OutDataTypeStr=Inherit: Same as first input
  Product7 : Product  Inputs=3  SaturateOnIntegerOverflow=on  InputSameDT=on  OutDataTypeStr=Inherit: Same as first input
  Sum1 : Sum  Inputs=-+  SaturateOnIntegerOverflow=on  InputSameDT=on  OutDataTypeStr=Inherit: Same as first input
  Switch : Switch  Criteria=u2 > Threshold
  Switch1 : Switch  Criteria=u2 > Threshold
  cp : Constant  Value=1006.8
  h/s : Gain  Gain=1/3600
  "[S]_in" : Outport
  "[S]_out" : Outport  Port=2
  wires:
  Mux3/1 -> Switch1/1
  Mux6/1 -> Switch1/3
  Bus Selector1/3 -> Fcn3/1  "<x_CO2>"
  Bus Selector1/2 -> Fcn4/1  "<x_H2O>"
  Fcn3/1 -> Mux3/2
  Fcn4/1 -> Mux3/1
  Bus Selector2/4 -> Switch/3  "<rho>"
  Bus Selector1/4 -> Switch/1  "<rho>"
  "[AIB]_in"/1 -> Bus Selector1/1
  cp/1 -> Product7/3
  Ground4/1 -> Mux1/7
  Ground1/1 -> Mux1/8
  "[AIB]_out"/1 -> Bus Selector2/1
  Bus Selector1/1 -> Sum1/1  "<Tc>"
  Fcn1/1 -> Mux6/2
  Fcn2/1 -> Mux6/1
  Ground12/1 -> Mux1/6
  Product5/1 -> Demux5/1
  Bus Selector2/3 -> Fcn1/1  "<x_CO2>"
  Mux2/1 -> "[S]_out"/1
  Switch/1 -> Product6/2  "rho"
  Product6/1 -> Gain1/1
  Gain/1 -> Switch/2, Switch1/2, h/s/1
  Mux1/1 -> "[S]_in"/1
  Product7/1 -> Gain2/1, Mux1/1  "Qdot_air"
  Ground13/1 -> Mux1/2
  Demux5/2 -> Mux1/5, Gain5/1  "mdot_CO2"
  Demux5/1 -> Mux1/4, Gain4/1  "mdot_H2O"
  Bus Selector2/1 -> Sum1/2  "<Tc>"
  Bus Selector2/2 -> Fcn2/1  "<x_H2O>"
  Switch1/1 -> Product5/2
  Sum1/1 -> Product7/1  "dT"
  Vdot/1 -> Gain/1
  h/s/1 -> Product6/1
  Gain1/1 -> Gain7/1, Product5/1, Product7/2, Mux1/3  "massflow"
  Ground3/1 -> Mux2/7
  Gain4/1 -> Mux2/4
  Gain7/1 -> Mux2/3
  Ground2/1 -> Mux2/2
  Gain5/1 -> Mux2/5
  Ground5/1 -> Mux2/6
  Ground6/1 -> Mux2/8
  Gain2/1 -> Mux2/1

== system building_EXAMPLE_v1/HVAC pipes/ventilation_zone-to-zone 1-9 ==
  "[AIB]_in" : Inport
  "[AIB]_out" : Inport  Port=2
  Vdot : Inport  Port=3
  Bus Selector1 : BusSelector  OutputSignals=Tc,x_H2O,x_CO2,rho
  Bus Selector2 : BusSelector  OutputSignals=Tc,x_H2O,x_CO2,rho
  Demux5 : Demux  Outputs=2
  Fcn{1..4} (4 alike) : Fcn  Expr=u / (1+u)
  Gain : Gain  Gain=perc_Vdot_tot
  Gain{1,4..5,7} (4 alike) : Gain  Gain=-1
  Gain2 : Gain  Gain=0
  Ground{1..6,12..13} (8 alike) : Ground
  Mux1 : Mux  Inputs=[1 2 1 1 1 5 1 7]
  Mux2 : Mux  Inputs=[1 2 1 1 1 5 1 7]
  Mux3 : Mux  Inputs=2
  Mux6 : Mux  Inputs=2
  Product5 : Product  SaturateOnIntegerOverflow=on  InputSameDT=on  OutDataTypeStr=Inherit: Same as first input
  Product6 : Product  SaturateOnIntegerOverflow=on  InputSameDT=on  OutDataTypeStr=Inherit: Same as first input
  Product7 : Product  Inputs=3  SaturateOnIntegerOverflow=on  InputSameDT=on  OutDataTypeStr=Inherit: Same as first input
  Sum1 : Sum  Inputs=-+  SaturateOnIntegerOverflow=on  InputSameDT=on  OutDataTypeStr=Inherit: Same as first input
  Switch : Switch  Criteria=u2 > Threshold
  Switch1 : Switch  Criteria=u2 > Threshold
  cp : Constant  Value=1006.8
  h/s : Gain  Gain=1/3600
  "[S]_in" : Outport
  "[S]_out" : Outport  Port=2
  wires:
  Mux3/1 -> Switch1/1
  Mux6/1 -> Switch1/3
  Bus Selector1/3 -> Fcn3/1  "<x_CO2>"
  Bus Selector1/2 -> Fcn4/1  "<x_H2O>"
  Fcn3/1 -> Mux3/2
  Fcn4/1 -> Mux3/1
  Bus Selector2/4 -> Switch/3  "<rho>"
  Bus Selector1/4 -> Switch/1  "<rho>"
  "[AIB]_in"/1 -> Bus Selector1/1
  cp/1 -> Product7/3
  Ground4/1 -> Mux1/7
  Ground1/1 -> Mux1/8
  "[AIB]_out"/1 -> Bus Selector2/1
  Bus Selector1/1 -> Sum1/1  "<Tc>"
  Fcn1/1 -> Mux6/2
  Fcn2/1 -> Mux6/1
  Ground12/1 -> Mux1/6
  Product5/1 -> Demux5/1
  Bus Selector2/3 -> Fcn1/1  "<x_CO2>"
  Mux2/1 -> "[S]_out"/1
  Switch/1 -> Product6/2  "rho"
  Product6/1 -> Gain1/1
  Gain/1 -> Switch/2, Switch1/2, h/s/1
  Mux1/1 -> "[S]_in"/1
  Product7/1 -> Gain2/1, Mux1/1  "Qdot_air"
  Ground13/1 -> Mux1/2
  Demux5/2 -> Mux1/5, Gain5/1  "mdot_CO2"
  Demux5/1 -> Mux1/4, Gain4/1  "mdot_H2O"
  Bus Selector2/1 -> Sum1/2  "<Tc>"
  Bus Selector2/2 -> Fcn2/1  "<x_H2O>"
  Switch1/1 -> Product5/2
  Sum1/1 -> Product7/1  "dT"
  Vdot/1 -> Gain/1
  h/s/1 -> Product6/1
  Gain1/1 -> Gain7/1, Product5/1, Product7/2, Mux1/3  "massflow"
  Ground3/1 -> Mux2/7
  Gain4/1 -> Mux2/4
  Gain7/1 -> Mux2/3
  Ground2/1 -> Mux2/2
  Gain5/1 -> Mux2/5
  Ground5/1 -> Mux2/6
  Ground6/1 -> Mux2/8
  Gain2/1 -> Mux2/1

== system building_EXAMPLE_v1/HVAC pipes/ventilation_zone-to-zone 2-10 ==
  "[AIB]_in" : Inport
  "[AIB]_out" : Inport  Port=2
  Vdot : Inport  Port=3
  Bus Selector1 : BusSelector  OutputSignals=Tc,x_H2O,x_CO2,rho
  Bus Selector2 : BusSelector  OutputSignals=Tc,x_H2O,x_CO2,rho
  Demux5 : Demux  Outputs=2
  Fcn{1..4} (4 alike) : Fcn  Expr=u / (1+u)
  Gain : Gain  Gain=perc_Vdot_tot
  Gain{1,4..5,7} (4 alike) : Gain  Gain=-1
  Gain2 : Gain  Gain=0
  Ground{1..6,12..13} (8 alike) : Ground
  Mux1 : Mux  Inputs=[1 2 1 1 1 5 1 7]
  Mux2 : Mux  Inputs=[1 2 1 1 1 5 1 7]
  Mux3 : Mux  Inputs=2
  Mux6 : Mux  Inputs=2
  Product5 : Product  SaturateOnIntegerOverflow=on  InputSameDT=on  OutDataTypeStr=Inherit: Same as first input
  Product6 : Product  SaturateOnIntegerOverflow=on  InputSameDT=on  OutDataTypeStr=Inherit: Same as first input
  Product7 : Product  Inputs=3  SaturateOnIntegerOverflow=on  InputSameDT=on  OutDataTypeStr=Inherit: Same as first input
  Sum1 : Sum  Inputs=-+  SaturateOnIntegerOverflow=on  InputSameDT=on  OutDataTypeStr=Inherit: Same as first input
  Switch : Switch  Criteria=u2 > Threshold
  Switch1 : Switch  Criteria=u2 > Threshold
  cp : Constant  Value=1006.8
  h/s : Gain  Gain=1/3600
  "[S]_in" : Outport
  "[S]_out" : Outport  Port=2
  wires:
  Mux3/1 -> Switch1/1
  Mux6/1 -> Switch1/3
  Bus Selector1/3 -> Fcn3/1  "<x_CO2>"
  Bus Selector1/2 -> Fcn4/1  "<x_H2O>"
  Fcn3/1 -> Mux3/2
  Fcn4/1 -> Mux3/1
  Bus Selector2/4 -> Switch/3  "<rho>"
  Bus Selector1/4 -> Switch/1  "<rho>"
  "[AIB]_in"/1 -> Bus Selector1/1
  cp/1 -> Product7/3
  Ground4/1 -> Mux1/7
  Ground1/1 -> Mux1/8
  "[AIB]_out"/1 -> Bus Selector2/1
  Bus Selector1/1 -> Sum1/1  "<Tc>"
  Fcn1/1 -> Mux6/2
  Fcn2/1 -> Mux6/1
  Ground12/1 -> Mux1/6
  Product5/1 -> Demux5/1
  Bus Selector2/3 -> Fcn1/1  "<x_CO2>"
  Mux2/1 -> "[S]_out"/1
  Switch/1 -> Product6/2  "rho"
  Product6/1 -> Gain1/1
  Gain/1 -> Switch/2, Switch1/2, h/s/1
  Mux1/1 -> "[S]_in"/1
  Product7/1 -> Gain2/1, Mux1/1  "Qdot_air"
  Ground13/1 -> Mux1/2
  Demux5/2 -> Mux1/5, Gain5/1  "mdot_CO2"
  Demux5/1 -> Mux1/4, Gain4/1  "mdot_H2O"
  Bus Selector2/1 -> Sum1/2  "<Tc>"
  Bus Selector2/2 -> Fcn2/1  "<x_H2O>"
  Switch1/1 -> Product5/2
  Sum1/1 -> Product7/1  "dT"
  Vdot/1 -> Gain/1
  h/s/1 -> Product6/1
  Gain1/1 -> Gain7/1, Product5/1, Product7/2, Mux1/3  "massflow"
  Ground3/1 -> Mux2/7
  Gain4/1 -> Mux2/4
  Gain7/1 -> Mux2/3
  Ground2/1 -> Mux2/2
  Gain5/1 -> Mux2/5
  Ground5/1 -> Mux2/6
  Ground6/1 -> Mux2/8
  Gain2/1 -> Mux2/1
